simulink model "globalSystemModel"  (R2021a)
settings: Solver=VariableStepAuto  StartTime=0.0  StopTime=10.0  RelTol=1e-3
values from neighbouring files (symbols this model uses):
  A = [A; A_i]    [Network.m]    (also in Subsystem.m = obj.A{obj.index}; jPaperData1.mat = [7.21225729966 1.39049686205 0 0 -0.282509513675 -0.19440187; jPaperData2.mat = [1.59283418225 -1.98990334273 -0.0774022354425 0.03883188575; paperData.mat = [-0.897343897753 -1.03363634124 0 0 0 0 -1.03363634124 -1.19)
  AcDiss =     [jPaperData1.mat]    (also in jPaperData2.mat)
  AcStab =     [jPaperData1.mat]    (also in jPaperData2.mat = [-4.66639923531 0.0224905641012 0.183856829633 -0.0600919958)
  B = [B; B_i]    [Network.m]    (also in Subsystem.m = obj.B{obj.index}; jPaperData1.mat = [0.133289291835 -2.25582289472 0 0 0 0 0 0 0 0 0 0 ... (50 e; jPaperData2.mat = [0.884783010265 -0.0578061269532 0 0 0 0 0 0 0 0 0 0 ... (50; paperData.mat = [-0.767652209467 0.0479827696564 0 0 0 0 0 0 0 0.69770450426)
  BcDiss =     [jPaperData1.mat]    (also in jPaperData2.mat)
  BcStab =     [jPaperData1.mat]    (also in jPaperData2.mat = [4.69331758427 -3.97574466957 -0.18243601768 0.0596281142245)
  C = [C; C_i]    [Network.m]    (also in Subsystem.m = {}; jPaperData1.mat = [-0.398868811937 0 0 0 0 0.199769403633 0 0 0 0 0 0 ... (50 ; jPaperData2.mat = [-2.29277321488 0 0 0 0 1.99520966434 0 0 0 0 0 0.4731154890; paperData.mat = [-0.192732954692 0 0 0.794595441386 0 0 0 1.44304729411 0 0 )
  CcDiss =     [jPaperData1.mat]    (also in jPaperData2.mat)
  CcStab =     [jPaperData1.mat]    (also in jPaperData2.mat = [3.40584102634 0.0670370876354 0 -0.466213574125 0.023320064)
  D = [D; D_i]    [Network.m]    (also in Subsystem.m = {}; jPaperData1.mat = [0 0 0 0 0 0 0 0 0 0 0 0 ... (25 elements, 5x5)]; jPaperData2.mat = [0 0 0 0 0 0 0 0 0 0 0 0 ... (25 elements, 5x5)]; paperData.mat = [0  0  0; 0  0  0; 0  0  0])
  DcDiss =     [jPaperData1.mat]    (also in jPaperData2.mat)
  DcStab =     [jPaperData1.mat]    (also in jPaperData2.mat = [-0.559949680356 -0.0227155093389 0 0.0369895329508 0.048553)
  E = [E; E_i]    [Network.m]    (also in Subsystem.m = {}; jPaperData1.mat = [0.013736298283 0.0126277412194 0 0 0 -0.00335268402912 0 0.; jPaperData2.mat = [-0.000849733283809 -0.00431479261265 0.00356522747973 0.001; paperData.mat = [0 0.622727541957 0 0 0 0 -0.10315996141 -0.125734072536 0 -)
  F = [F; F_i]    [Network.m]    (also in Subsystem.m = {}; jPaperData1.mat = [0 0 0 0 0 0 0.00667542601126 0 0 0 0 0 ... (25 elements, 5x; jPaperData2.mat = [0 0 0 0 0 0 0 0 0 0 0 0 ... (25 elements, 5x5)]; paperData.mat = [0.160906008337  0  0; 0  0.0149076612258  0; 0  0  0])
  G = [1 0 0 0 0 1 0 0 0 0 0 1 ... (50 elements, 5x10)]    [jPaperData1.mat]    (also in jPaperData2.mat)
  H = [1 0 0 0 0 0 1 0 0 0 0 0 ... (25 elements, 5x5)]    [jPaperData1.mat]    (also in jPaperData2.mat)
  J = [1 0 0 0 0 0 1 0 0 0 0 0 ... (25 elements, 5x5)]    [jPaperData1.mat]    (also in jPaperData2.mat)
  KDiss = [0 0 0 0 0 0 0 0 0 0 0 0 ... (50 elements, 5x10)]    [jPaperData1.mat]    (also in jPaperData2.mat)
  KStab =     [jPaperData1.mat]    (also in jPaperData2.mat = [-4.86369493868 -0.00198336219621 0 -0.960462012264 -0.04588)
  LDiss =     [jPaperData1.mat]    (also in jPaperData2.mat = [-3.49678545473 -0.771253400681 0.0276218519768 -0.070221237)
  LStab =     [jPaperData1.mat]    (also in jPaperData2.mat = [-2.23296914639 -0.236331029549 0.0275982481338 -0.070133150)
  n = obj.dim_n    [Subsystem.m]    (also in jPaperData1.mat = 10; jPaperData2.mat = 10; temp1.m = size(A,1); temp10.m = 4)
libraries: simulink x1
settings Model: Creator=Shirantha Welikala  LastModifiedBy=Shirantha Welikala

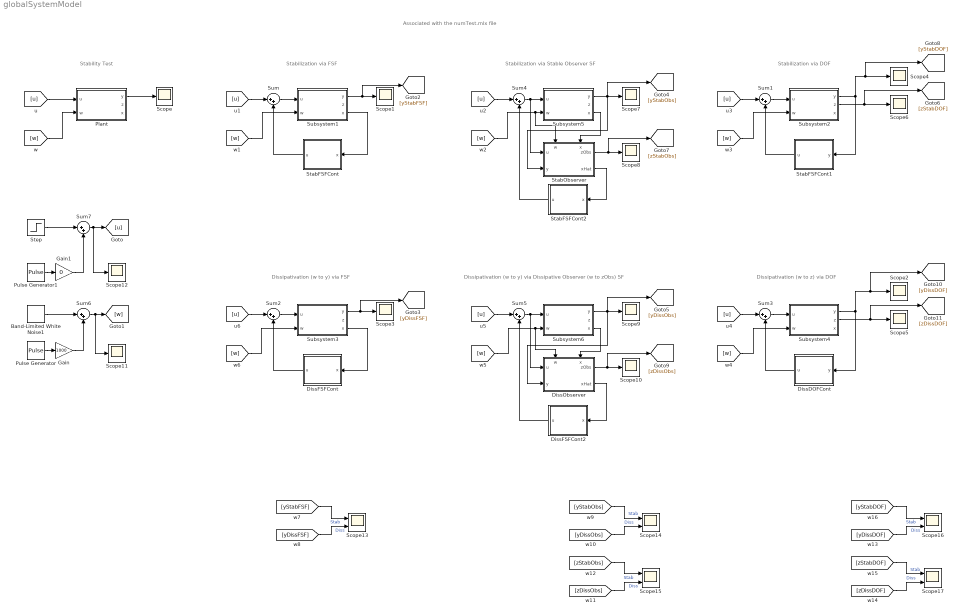
== system globalSystemModel ==
  note: Associated with the numTest.mlx file
  note: Stability Test
  note: Stabilization via FSF
  note: Stabilization via DOF
  note: Dissipativation (w to y) via FSF
  note: Dissipativation (w to z) via DOF
  note: Stabilization via Stable Observer SF
  note: Dissipativation (w to y) via Dissipative Observer (w to zObs) SF
  Band-Limited White Noise1 : simulink/Sources/Band-Limited White Noise  Cov=[1]  Ts=0.01  seed=[23341]
  DissDOFCont : Subsystem
  DissFSFCont : Subsystem
  DissFSFCont2 : Subsystem
  DissObserver : Subsystem
      settings: PortSchema="{\"entries\":[{\"content\":{\"sides\":[{\"content\":{\"connectorIds\":[\"In1\",\"In2\"]},\"type\":\"ConnectorPlacement.EquallySpacedRectSide\",\"uuid\":\"bb89ae44-d021-4487-97ea-d884edbfbdc6\"},{\"content\":{\"connectorIds\":[\"Out1\",\"Out2\"],\"side\":\"RIGHT\"},\"type\":\"ConnectorPlacement.EquallySpacedRectSide\",\"uuid\":\"8b439939-30ad-482f-a8e7-d460793e5232\"},{\"content\":{\"connectorIds\":[\"In3\",\"In4\"],\"side\":\"TOP\"},\"type\":\"ConnectorPlacement.EquallySpacedRectSide\",\"uuid\":\"831faa58-2099-4155-89c8-01b636ce25d5\"}]},\"type\":\"ConnectorPlacement.EquallySpacedConnector\",\"uuid\":\"0a775592-9d3b-4995-aaad-fe94d15f27f2\"}],\"packageUris\":[\"http://schema.mathworks.com/mf0/Connector/R2020b\"],\"version\":\"1.0\"}"
  Gain : Gain  Gain=1000
  Gain1 : Gain  Gain=0
  Plant : Subsystem
  Pulse Generator : DiscretePulseGenerator  PulseType=Time based  Period=10  PhaseDelay=5
  Pulse Generator1 : DiscretePulseGenerator  PulseType=Time based  Period=10  PulseWidth=10  PhaseDelay=5
  Scope{,1..12} (13 alike) : Scope
  Scope{13..17} (5 alike) : Scope  NumInputPorts=2
  StabFSFCont : Subsystem
  StabFSFCont1 : Subsystem
  StabFSFCont2 : Subsystem
  StabObserver : Subsystem
      settings: PortSchema="{\"entries\":[{\"content\":{\"sides\":[{\"content\":{\"connectorIds\":[\"In1\",\"In2\"]},\"type\":\"ConnectorPlacement.EquallySpacedRectSide\",\"uuid\":\"bb89ae44-d021-4487-97ea-d884edbfbdc6\"},{\"content\":{\"connectorIds\":[\"Out1\",\"Out2\"],\"side\":\"RIGHT\"},\"type\":\"ConnectorPlacement.EquallySpacedRectSide\",\"uuid\":\"8b439939-30ad-482f-a8e7-d460793e5232\"},{\"content\":{\"connectorIds\":[\"In3\",\"In4\"],\"side\":\"TOP\"},\"type\":\"ConnectorPlacement.EquallySpacedRectSide\",\"uuid\":\"831faa58-2099-4155-89c8-01b636ce25d5\"}]},\"type\":\"ConnectorPlacement.EquallySpacedConnector\",\"uuid\":\"0a775592-9d3b-4995-aaad-fe94d15f27f2\"}],\"packageUris\":[\"http://schema.mathworks.com/mf0/Connector/R2020b\"],\"version\":\"1.0\"}"
  Step : Step  SampleTime=0
  Subsystem1 : Subsystem
  Subsystem2 : Subsystem
  Subsystem3 : Subsystem
  Subsystem4 : Subsystem
  Subsystem5 : Subsystem
  Subsystem6 : Subsystem
  Sum{,1..7} (8 alike) : Sum  Inputs=|++
  wires:
  Plant/1(y) -> Scope/1
  [u] -> Plant/1(u)
  Subsystem1/1(y) -> [yStabFSF], Scope1/1
  Subsystem1/3(x) -> StabFSFCont/1(x)
  [u] -> Sum/1
  Sum/1 -> Subsystem1/1(u)
  StabFSFCont1/1(u) -> Sum1/2
  Subsystem2/1(y) -> [yStabDOF], Scope4/1, StabFSFCont1/1(y)
  Sum1/1 -> Subsystem2/1(u)
  [w] -> Subsystem1/2(w)
  [w] -> Plant/2(w)
  StabFSFCont/1(u) -> Sum/2
  Subsystem3/1(y) -> [yDissFSF], Scope3/1
  Subsystem3/3(x) -> DissFSFCont/1(x)
  [u] -> Sum2/1
  Sum2/1 -> Subsystem3/1(u)
  DissFSFCont/1(u) -> Sum2/2
  Sum3/1 -> Subsystem4/1(u)
  [u] -> Sum3/1
  DissDOFCont/1(u) -> Sum3/2
  Subsystem4/1(y) -> DissDOFCont/1(y), Scope2/1, [yDissDOF]
  Subsystem4/2(z) -> [zDissDOF], Scope5/1
  Subsystem2/2(z) -> [zStabDOF], Scope6/1
  Sum4/1 -> StabObserver/1(u), Subsystem5/1(u)
  StabFSFCont2/1(u) -> Sum4/2
  Subsystem5/3(x) -> StabObserver/4(x)
  Subsystem5/1(y) -> Scope7/1, [yStabObs], StabObserver/2(y)
  StabObserver/1(zObs) -> [zStabObs], Scope8/1
  StabObserver/2(xHat) -> StabFSFCont2/1(x)
  DissObserver/2(xHat) -> DissFSFCont2/1(x)
  DissObserver/1(zObs) -> [zDissObs], Scope10/1
  Subsystem6/3(x) -> DissObserver/4(x)
  Sum5/1 -> DissObserver/1(u), Subsystem6/1(u)
  DissFSFCont2/1(u) -> Sum5/2
  Subsystem6/1(y) -> [yDissObs], DissObserver/2(y), Scope9/1
  [w] -> DissObserver/3(w), Subsystem6/2(w)
  Band-Limited White Noise1/1 -> Sum6/1
  Sum6/1 -> Scope11/1, [w]
  Gain/1 -> Sum6/2
  Pulse Generator/1 -> Gain/1
  Gain1/1 -> Sum7/2
  Sum7/1 -> Scope12/1, [u]
  Pulse Generator1/1 -> Gain1/1
  Step/1 -> Sum7/1
  [u] -> Sum4/1
  [w] -> StabObserver/3(w), Subsystem5/2(w)
  [w] -> Subsystem3/2(w)
  [u] -> Sum5/1
  [w] -> Subsystem4/2(w)
  [u] -> Sum1/1
  [w] -> Subsystem2/2(w)
  [yStabFSF] -> Scope13/1  "Stab"
  [yDissFSF] -> Scope13/2  "Diss"
  [yDissObs] -> Scope14/2  "Diss"
  [yStabObs] -> Scope14/1  "Stab"
  [zStabObs] -> Scope15/1  "Stab"
  [zDissObs] -> Scope15/2  "Diss"
  [yStabDOF] -> Scope16/1  "Stab"
  [zDissDOF] -> Scope17/2  "Diss"
  [zStabDOF] -> Scope17/1  "Stab"
  [yDissDOF] -> Scope16/2  "Diss"

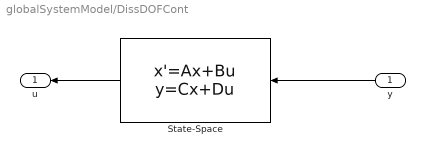
== system globalSystemModel/DissDOFCont ==
  y : Inport
  State-Space : StateSpace  A=AcDiss  B=BcDiss  C=CcDiss  D=DcDiss  InitialCondition=zeros(n,1)
  u : Outport
  wires:
  y/1 -> State-Space/1
  State-Space/1 -> u/1

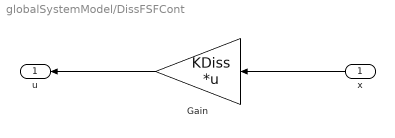
== system globalSystemModel/DissFSFCont ==
  x : Inport
  Gain : Gain  Gain=KDiss  Multiplication=Matrix(K*u)
  u : Outport
  wires:
  x/1 -> Gain/1
  Gain/1 -> u/1

== system globalSystemModel/DissFSFCont2 ==
  x : Inport
  Gain : Gain  Gain=KDiss  Multiplication=Matrix(K*u)
  u : Outport
  wires:
  x/1 -> Gain/1
  Gain/1 -> u/1

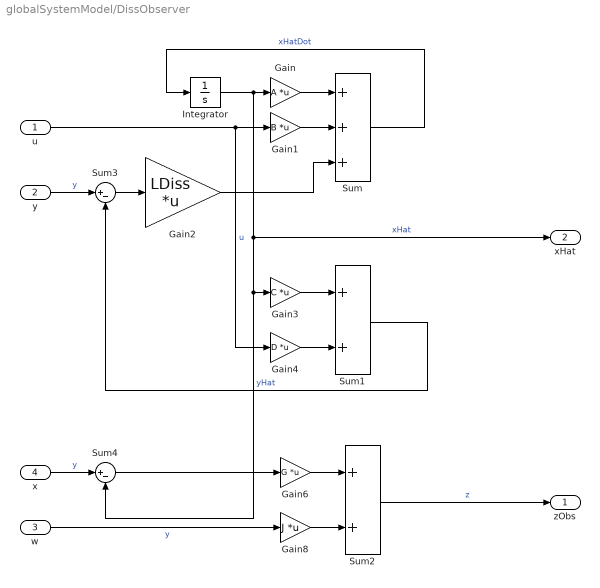
== system globalSystemModel/DissObserver ==
  u : Inport
  y : Inport  Port=2
  w : Inport  Port=3
  x : Inport  Port=4
  Gain : Gain  Gain=A  Multiplication=Matrix(K*u)
  Gain1 : Gain  Gain=B  Multiplication=Matrix(K*u)
  Gain2 : Gain  Gain=LDiss  Multiplication=Matrix(K*u)
  Gain3 : Gain  Gain=C  Multiplication=Matrix(K*u)
  Gain4 : Gain  Gain=D  Multiplication=Matrix(K*u)
  Gain6 : Gain  Gain=G  Multiplication=Matrix(K*u)
  Gain8 : Gain  Gain=J  Multiplication=Matrix(K*u)
  Integrator : Integrator  InitialCondition=zeros(n,1)
  Sum : Sum  Inputs=+++
  Sum1 : Sum
  Sum2 : Sum
  Sum3 : Sum  Inputs=|+-
  Sum4 : Sum  Inputs=|+-
  zObs : Outport
  xHat : Outport  Port=2
  wires:
  Gain2/1 -> Sum/3
  Sum/1 -> Integrator/1  "xHatDot"
  Gain/1 -> Sum/1
  Gain1/1 -> Sum/2
  Integrator/1 -> Sum4/2, Gain3/1, xHat/1, Gain/1  "xHat"
  Sum2/1 -> zObs/1  "z"
  Gain8/1 -> Sum2/2
  Gain6/1 -> Sum2/1
  u/1 -> Gain1/1, Gain4/1  "u"
  Gain4/1 -> Sum1/2
  Sum1/1 -> Sum3/2  "yHat"
  Gain3/1 -> Sum1/1
  y/1 -> Sum3/1  "y"
  Sum3/1 -> Gain2/1
  x/1 -> Sum4/1  "y"
  Sum4/1 -> Gain6/1
  w/1 -> Gain8/1  "y"

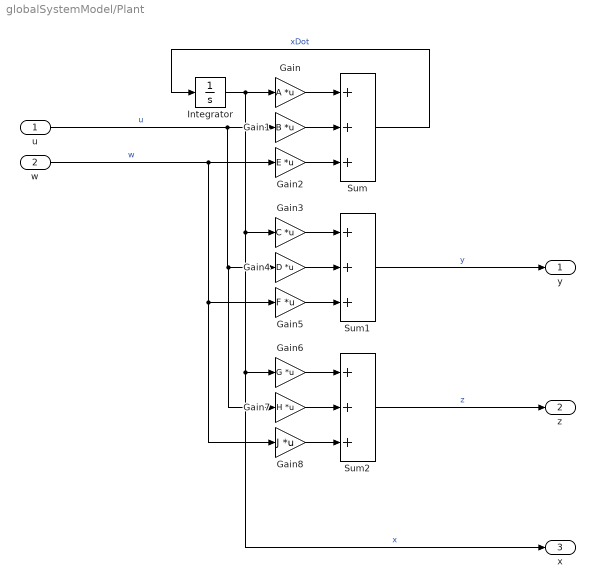
== system globalSystemModel/Plant ==
  u : Inport
  w : Inport  Port=2
  Gain : Gain  Gain=A  Multiplication=Matrix(K*u)
  Gain1 : Gain  Gain=B  Multiplication=Matrix(K*u)
  Gain2 : Gain  Gain=E  Multiplication=Matrix(K*u)
  Gain3 : Gain  Gain=C  Multiplication=Matrix(K*u)
  Gain4 : Gain  Gain=D  Multiplication=Matrix(K*u)
  Gain5 : Gain  Gain=F  Multiplication=Matrix(K*u)
  Gain6 : Gain  Gain=G  Multiplication=Matrix(K*u)
  Gain7 : Gain  Gain=H  Multiplication=Matrix(K*u)
  Gain8 : Gain  Gain=J  Multiplication=Matrix(K*u)
  Integrator : Integrator  InitialCondition=10*ones(n,1)
  Sum : Sum  Inputs=+++
  Sum1 : Sum  Inputs=+++
  Sum2 : Sum  Inputs=+++
  y : Outport
  z : Outport  Port=2
  x : Outport  Port=3
  wires:
  u/1 -> Gain7/1, Gain4/1, Gain1/1  "u"
  Gain2/1 -> Sum/3
  w/1 -> Gain8/1, Gain5/1, Gain2/1  "w"
  Gain3/1 -> Sum1/1
  Sum/1 -> Integrator/1  "xDot"
  Gain5/1 -> Sum1/3
  Gain/1 -> Sum/1
  Gain1/1 -> Sum/2
  Gain4/1 -> Sum1/2
  Sum2/1 -> z/1  "z"
  Sum1/1 -> y/1  "y"
  Gain8/1 -> Sum2/3
  Gain6/1 -> Sum2/1
  Gain7/1 -> Sum2/2
  Integrator/1 -> x/1, Gain6/1, Gain3/1, Gain/1  "x"

== system globalSystemModel/StabFSFCont ==
  x : Inport
  Gain : Gain  Gain=KStab  Multiplication=Matrix(K*u)
  u : Outport
  wires:
  x/1 -> Gain/1
  Gain/1 -> u/1

== system globalSystemModel/StabFSFCont1 ==
  y : Inport
  State-Space : StateSpace  A=AcStab  B=BcStab  C=CcStab  D=DcStab  InitialCondition=zeros(n,1)
  u : Outport
  wires:
  y/1 -> State-Space/1
  State-Space/1 -> u/1

== system globalSystemModel/StabFSFCont2 ==
  x : Inport
  Gain : Gain  Gain=KStab  Multiplication=Matrix(K*u)
  u : Outport
  wires:
  x/1 -> Gain/1
  Gain/1 -> u/1

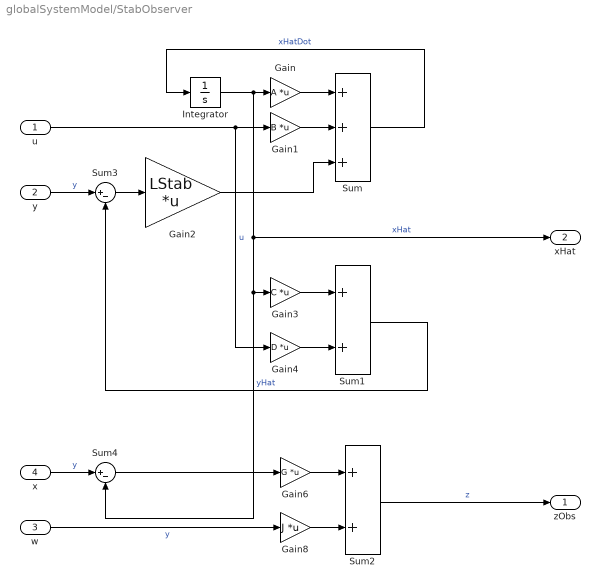
== system globalSystemModel/StabObserver ==
  u : Inport
  y : Inport  Port=2
  w : Inport  Port=3
  x : Inport  Port=4
  Gain : Gain  Gain=A  Multiplication=Matrix(K*u)
  Gain1 : Gain  Gain=B  Multiplication=Matrix(K*u)
  Gain2 : Gain  Gain=LStab  Multiplication=Matrix(K*u)
  Gain3 : Gain  Gain=C  Multiplication=Matrix(K*u)
  Gain4 : Gain  Gain=D  Multiplication=Matrix(K*u)
  Gain6 : Gain  Gain=G  Multiplication=Matrix(K*u)
  Gain8 : Gain  Gain=J  Multiplication=Matrix(K*u)
  Integrator : Integrator  InitialCondition=zeros(n,1)
  Sum : Sum  Inputs=+++
  Sum1 : Sum
  Sum2 : Sum
  Sum3 : Sum  Inputs=|+-
  Sum4 : Sum  Inputs=|+-
  zObs : Outport
  xHat : Outport  Port=2
  wires:
  Gain2/1 -> Sum/3
  Sum/1 -> Integrator/1  "xHatDot"
  Gain/1 -> Sum/1
  Gain1/1 -> Sum/2
  Integrator/1 -> Sum4/2, Gain3/1, xHat/1, Gain/1  "xHat"
  Sum2/1 -> zObs/1  "z"
  Gain8/1 -> Sum2/2
  Gain6/1 -> Sum2/1
  u/1 -> Gain1/1, Gain4/1  "u"
  Gain4/1 -> Sum1/2
  Sum1/1 -> Sum3/2  "yHat"
  Gain3/1 -> Sum1/1
  y/1 -> Sum3/1  "y"
  Sum3/1 -> Gain2/1
  x/1 -> Sum4/1  "y"
  Sum4/1 -> Gain6/1
  w/1 -> Gain8/1  "y"

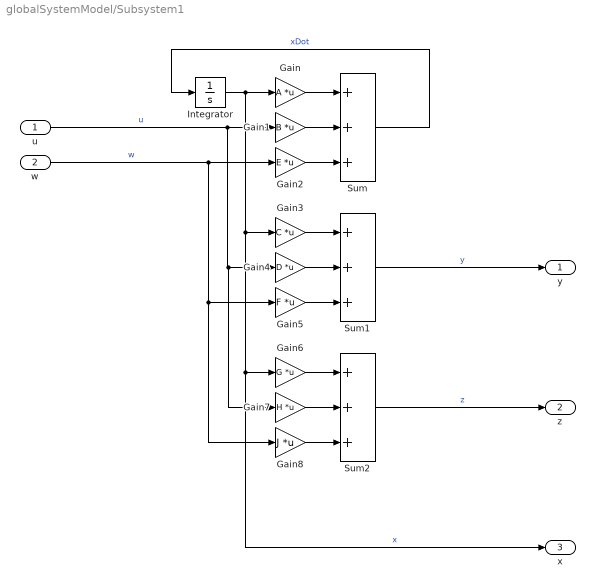
== system globalSystemModel/Subsystem1 ==
  u : Inport
  w : Inport  Port=2
  Gain : Gain  Gain=A  Multiplication=Matrix(K*u)
  Gain1 : Gain  Gain=B  Multiplication=Matrix(K*u)
  Gain2 : Gain  Gain=E  Multiplication=Matrix(K*u)
  Gain3 : Gain  Gain=C  Multiplication=Matrix(K*u)
  Gain4 : Gain  Gain=D  Multiplication=Matrix(K*u)
  Gain5 : Gain  Gain=F  Multiplication=Matrix(K*u)
  Gain6 : Gain  Gain=G  Multiplication=Matrix(K*u)
  Gain7 : Gain  Gain=H  Multiplication=Matrix(K*u)
  Gain8 : Gain  Gain=J  Multiplication=Matrix(K*u)
  Integrator : Integrator  InitialCondition=10*ones(n,1)
  Sum : Sum  Inputs=+++
  Sum1 : Sum  Inputs=+++
  Sum2 : Sum  Inputs=+++
  y : Outport
  z : Outport  Port=2
  x : Outport  Port=3
  wires:
  u/1 -> Gain7/1, Gain4/1, Gain1/1  "u"
  Gain2/1 -> Sum/3
  w/1 -> Gain8/1, Gain5/1, Gain2/1  "w"
  Gain3/1 -> Sum1/1
  Sum/1 -> Integrator/1  "xDot"
  Gain5/1 -> Sum1/3
  Gain/1 -> Sum/1
  Gain1/1 -> Sum/2
  Integrator/1 -> x/1, Gain6/1, Gain3/1, Gain/1  "x"
  Gain4/1 -> Sum1/2
  Sum2/1 -> z/1  "z"
  Sum1/1 -> y/1  "y"
  Gain8/1 -> Sum2/3
  Gain6/1 -> Sum2/1
  Gain7/1 -> Sum2/2

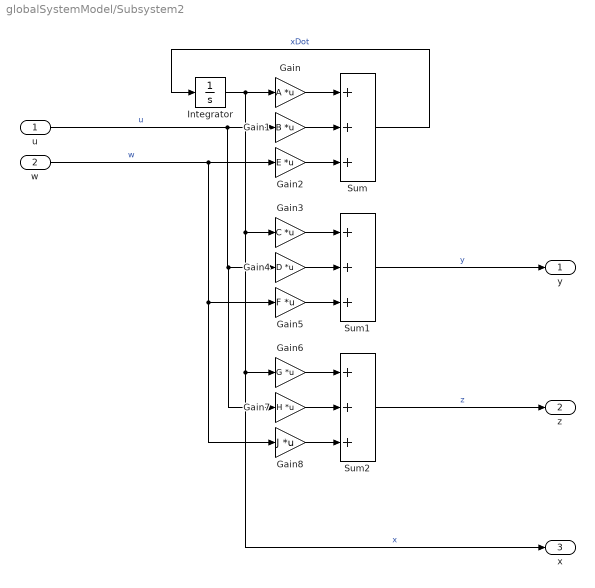
== system globalSystemModel/Subsystem2 ==
  u : Inport
  w : Inport  Port=2
  Gain : Gain  Gain=A  Multiplication=Matrix(K*u)
  Gain1 : Gain  Gain=B  Multiplication=Matrix(K*u)
  Gain2 : Gain  Gain=E  Multiplication=Matrix(K*u)
  Gain3 : Gain  Gain=C  Multiplication=Matrix(K*u)
  Gain4 : Gain  Gain=D  Multiplication=Matrix(K*u)
  Gain5 : Gain  Gain=F  Multiplication=Matrix(K*u)
  Gain6 : Gain  Gain=G  Multiplication=Matrix(K*u)
  Gain7 : Gain  Gain=H  Multiplication=Matrix(K*u)
  Gain8 : Gain  Gain=J  Multiplication=Matrix(K*u)
  Integrator : Integrator  InitialCondition=10*ones(n,1)
  Sum : Sum  Inputs=+++
  Sum1 : Sum  Inputs=+++
  Sum2 : Sum  Inputs=+++
  y : Outport
  z : Outport  Port=2
  x : Outport  Port=3
  wires:
  u/1 -> Gain7/1, Gain4/1, Gain1/1  "u"
  Gain2/1 -> Sum/3
  w/1 -> Gain8/1, Gain5/1, Gain2/1  "w"
  Gain3/1 -> Sum1/1
  Sum/1 -> Integrator/1  "xDot"
  Gain5/1 -> Sum1/3
  Gain/1 -> Sum/1
  Gain1/1 -> Sum/2
  Integrator/1 -> x/1, Gain6/1, Gain3/1, Gain/1  "x"
  Gain4/1 -> Sum1/2
  Sum2/1 -> z/1  "z"
  Sum1/1 -> y/1  "y"
  Gain8/1 -> Sum2/3
  Gain6/1 -> Sum2/1
  Gain7/1 -> Sum2/2

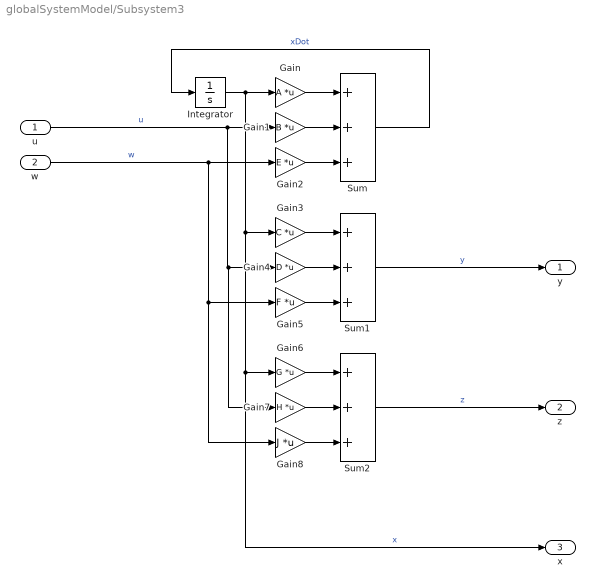
== system globalSystemModel/Subsystem3 ==
  u : Inport
  w : Inport  Port=2
  Gain : Gain  Gain=A  Multiplication=Matrix(K*u)
  Gain1 : Gain  Gain=B  Multiplication=Matrix(K*u)
  Gain2 : Gain  Gain=E  Multiplication=Matrix(K*u)
  Gain3 : Gain  Gain=C  Multiplication=Matrix(K*u)
  Gain4 : Gain  Gain=D  Multiplication=Matrix(K*u)
  Gain5 : Gain  Gain=F  Multiplication=Matrix(K*u)
  Gain6 : Gain  Gain=G  Multiplication=Matrix(K*u)
  Gain7 : Gain  Gain=H  Multiplication=Matrix(K*u)
  Gain8 : Gain  Gain=J  Multiplication=Matrix(K*u)
  Integrator : Integrator  InitialCondition=10*ones(n,1)
  Sum : Sum  Inputs=+++
  Sum1 : Sum  Inputs=+++
  Sum2 : Sum  Inputs=+++
  y : Outport
  z : Outport  Port=2
  x : Outport  Port=3
  wires:
  u/1 -> Gain7/1, Gain4/1, Gain1/1  "u"
  Gain2/1 -> Sum/3
  w/1 -> Gain8/1, Gain5/1, Gain2/1  "w"
  Gain3/1 -> Sum1/1
  Sum/1 -> Integrator/1  "xDot"
  Gain5/1 -> Sum1/3
  Gain/1 -> Sum/1
  Gain1/1 -> Sum/2
  Integrator/1 -> x/1, Gain6/1, Gain3/1, Gain/1  "x"
  Gain4/1 -> Sum1/2
  Sum2/1 -> z/1  "z"
  Sum1/1 -> y/1  "y"
  Gain8/1 -> Sum2/3
  Gain6/1 -> Sum2/1
  Gain7/1 -> Sum2/2

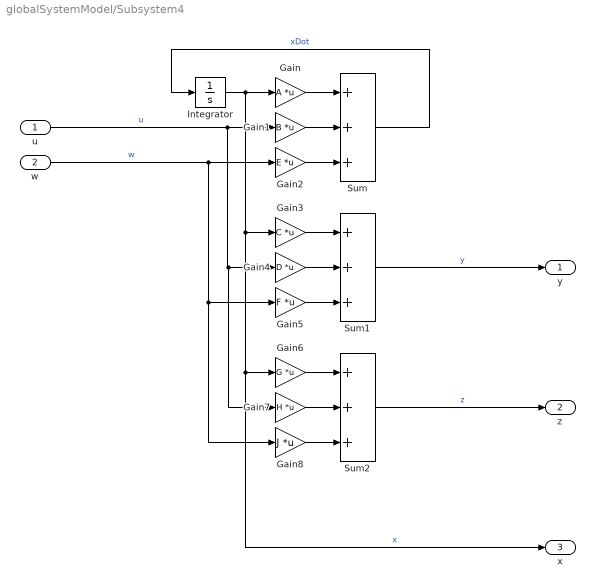
== system globalSystemModel/Subsystem4 ==
  u : Inport
  w : Inport  Port=2
  Gain : Gain  Gain=A  Multiplication=Matrix(K*u)
  Gain1 : Gain  Gain=B  Multiplication=Matrix(K*u)
  Gain2 : Gain  Gain=E  Multiplication=Matrix(K*u)
  Gain3 : Gain  Gain=C  Multiplication=Matrix(K*u)
  Gain4 : Gain  Gain=D  Multiplication=Matrix(K*u)
  Gain5 : Gain  Gain=F  Multiplication=Matrix(K*u)
  Gain6 : Gain  Gain=G  Multiplication=Matrix(K*u)
  Gain7 : Gain  Gain=H  Multiplication=Matrix(K*u)
  Gain8 : Gain  Gain=J  Multiplication=Matrix(K*u)
  Integrator : Integrator  InitialCondition=10*ones(n,1)
  Sum : Sum  Inputs=+++
  Sum1 : Sum  Inputs=+++
  Sum2 : Sum  Inputs=+++
  y : Outport
  z : Outport  Port=2
  x : Outport  Port=3
  wires:
  u/1 -> Gain7/1, Gain4/1, Gain1/1  "u"
  Gain2/1 -> Sum/3
  w/1 -> Gain8/1, Gain5/1, Gain2/1  "w"
  Gain3/1 -> Sum1/1
  Sum/1 -> Integrator/1  "xDot"
  Gain5/1 -> Sum1/3
  Gain/1 -> Sum/1
  Gain1/1 -> Sum/2
  Integrator/1 -> x/1, Gain6/1, Gain3/1, Gain/1  "x"
  Gain4/1 -> Sum1/2
  Sum2/1 -> z/1  "z"
  Sum1/1 -> y/1  "y"
  Gain8/1 -> Sum2/3
  Gain6/1 -> Sum2/1
  Gain7/1 -> Sum2/2

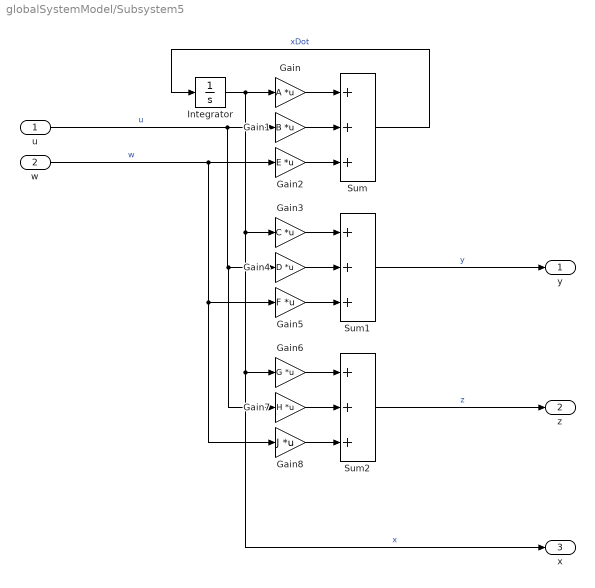
== system globalSystemModel/Subsystem5 ==
  u : Inport
  w : Inport  Port=2
  Gain : Gain  Gain=A  Multiplication=Matrix(K*u)
  Gain1 : Gain  Gain=B  Multiplication=Matrix(K*u)
  Gain2 : Gain  Gain=E  Multiplication=Matrix(K*u)
  Gain3 : Gain  Gain=C  Multiplication=Matrix(K*u)
  Gain4 : Gain  Gain=D  Multiplication=Matrix(K*u)
  Gain5 : Gain  Gain=F  Multiplication=Matrix(K*u)
  Gain6 : Gain  Gain=G  Multiplication=Matrix(K*u)
  Gain7 : Gain  Gain=H  Multiplication=Matrix(K*u)
  Gain8 : Gain  Gain=J  Multiplication=Matrix(K*u)
  Integrator : Integrator  InitialCondition=10*ones(n,1)
  Sum : Sum  Inputs=+++
  Sum1 : Sum  Inputs=+++
  Sum2 : Sum  Inputs=+++
  y : Outport
  z : Outport  Port=2
  x : Outport  Port=3
  wires:
  u/1 -> Gain7/1, Gain4/1, Gain1/1  "u"
  Gain2/1 -> Sum/3
  w/1 -> Gain8/1, Gain5/1, Gain2/1  "w"
  Gain3/1 -> Sum1/1
  Sum/1 -> Integrator/1  "xDot"
  Gain5/1 -> Sum1/3
  Gain/1 -> Sum/1
  Gain1/1 -> Sum/2
  Integrator/1 -> x/1, Gain6/1, Gain3/1, Gain/1  "x"
  Gain4/1 -> Sum1/2
  Sum2/1 -> z/1  "z"
  Sum1/1 -> y/1  "y"
  Gain8/1 -> Sum2/3
  Gain6/1 -> Sum2/1
  Gain7/1 -> Sum2/2

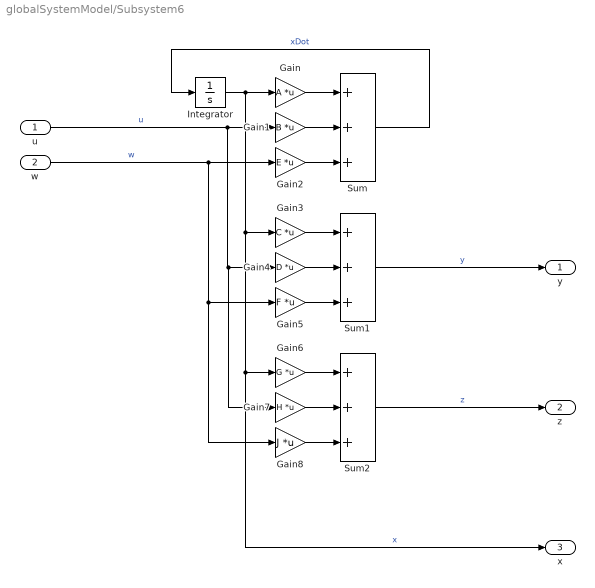
== system globalSystemModel/Subsystem6 ==
  u : Inport
  w : Inport  Port=2
  Gain : Gain  Gain=A  Multiplication=Matrix(K*u)
  Gain1 : Gain  Gain=B  Multiplication=Matrix(K*u)
  Gain2 : Gain  Gain=E  Multiplication=Matrix(K*u)
  Gain3 : Gain  Gain=C  Multiplication=Matrix(K*u)
  Gain4 : Gain  Gain=D  Multiplication=Matrix(K*u)
  Gain5 : Gain  Gain=F  Multiplication=Matrix(K*u)
  Gain6 : Gain  Gain=G  Multiplication=Matrix(K*u)
  Gain7 : Gain  Gain=H  Multiplication=Matrix(K*u)
  Gain8 : Gain  Gain=J  Multiplication=Matrix(K*u)
  Integrator : Integrator  InitialCondition=10*ones(n,1)
  Sum : Sum  Inputs=+++
  Sum1 : Sum  Inputs=+++
  Sum2 : Sum  Inputs=+++
  y : Outport
  z : Outport  Port=2
  x : Outport  Port=3
  wires:
  u/1 -> Gain7/1, Gain4/1, Gain1/1  "u"
  Gain2/1 -> Sum/3
  w/1 -> Gain8/1, Gain5/1, Gain2/1  "w"
  Gain3/1 -> Sum1/1
  Sum/1 -> Integrator/1  "xDot"
  Gain5/1 -> Sum1/3
  Gain/1 -> Sum/1
  Gain1/1 -> Sum/2
  Integrator/1 -> x/1, Gain6/1, Gain3/1, Gain/1  "x"
  Gain4/1 -> Sum1/2
  Sum2/1 -> z/1  "z"
  Sum1/1 -> y/1  "y"
  Gain8/1 -> Sum2/3
  Gain6/1 -> Sum2/1
  Gain7/1 -> Sum2/2
